simulink model "dyn_ESM_KF_SSM_VI_data"  (R2024b)
settings: Solver=ode1be  StartTime=0.0  StopTime=10  FixedStep=0.001  RelTol=1e-3
values from neighbouring files (symbols this model uses):
  A = [a11 a12; a21 a22]    [bicycleModelParam.m]
  B = [b1; b2]    [bicycleModelParam.m]
  H = [1 0;0 1]    [bicycleModelParam.m]
  Q = diag([0.2, 0.2, 0.01, 0.5, 0.3, 0.0001, 0.001, 0, 0.05])    [Copy_of_bicycleModelParam.m]    (also in bicycleModelParam.m = [0.8 0.2; 0.4 0.8])
  R = 0.001    [bicycleModelParam.m]
  v = 18/3.6    (= 5)    [bicycleModelParam.m]
libraries: simulink_extras x10
settings Model: Creator=fanny  LastModifiedBy=fanny
settings OptimizationCC: BlockReduction=off  DefaultParameterBehavior=Inlined  BufferReuse=off
settings DebuggingCC: AlgebraicLoopMsg=none

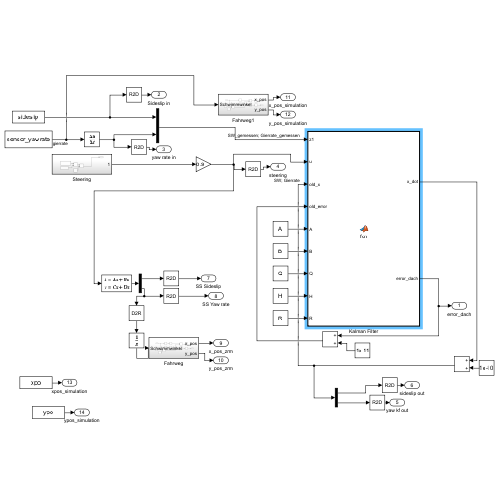
[thumbnail: Simulink's stored preview of the top-level diagram]
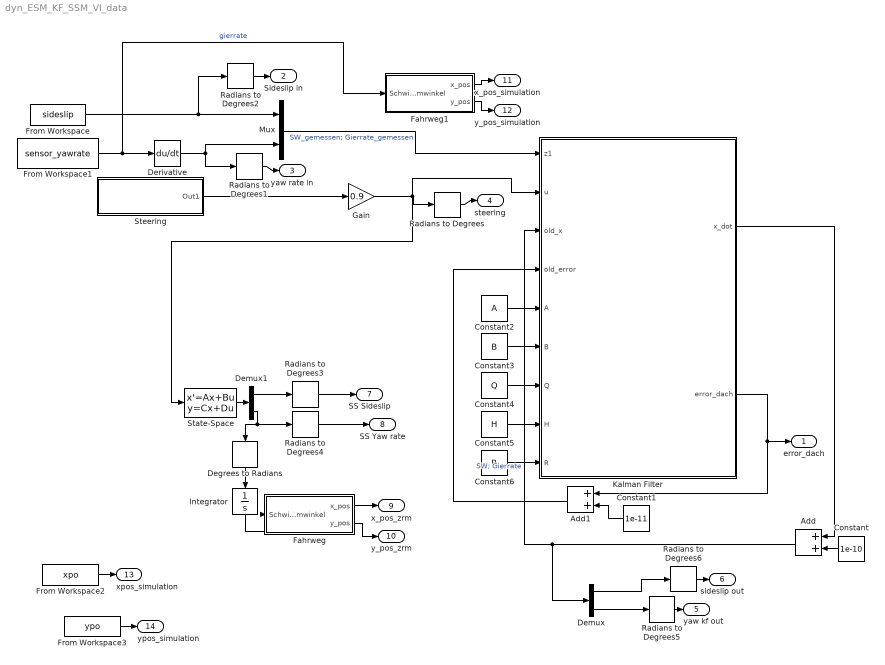
== system dyn_ESM_KF_SSM_VI_data ==
  Add : Sum
  Add1 : Sum
  Constant : Constant  Value=1e-10
  Constant1 : Constant  Value=1e-11
  Constant2 : Constant  Value=A
  Constant3 : Constant  Value=B
  Constant4 : Constant  Value=Q
  Constant5 : Constant  Value=H
  Constant6 : Constant  Value=R
  Degrees to Radians : simulink_extras/Transformations/Degrees to Radians
  Demux : Demux  Outputs=2
  Demux1 : Demux  Outputs=2
  Derivative : Derivative
  Fahrweg : Subsystem
  Fahrweg1 : Subsystem
  From Workspace : FromWorkspace  VariableName=sideslip
  From Workspace1 : FromWorkspace  VariableName=sensor_yawrate
  From Workspace2 : FromWorkspace  VariableName=xpo
  From Workspace3 : FromWorkspace  VariableName=ypo
  Gain : Gain  Gain=0.9
  Integrator : Integrator
  Kalman Filter : MATLAB Function  TreatAsAtomicUnit=on
  Mux : Mux  Inputs=2
  Radians to Degrees{,1..6} (7 alike) : simulink_extras/Transformations/Radians to Degrees
  State-Space : StateSpace  A=A  B=B  C=[1 0; 0 57]  D=[0; 0]  InitialCondition=0
  Steering : Subsystem
  error_dach : Outport
  Sideslip in : Outport  Port=2
  yaw rate in : Outport  Port=3
  steering : Outport  Port=4
  yaw kf out : Outport  Port=5
  sideslip out : Outport  Port=6
  SS Sideslip : Outport  Port=7
  SS Yaw rate : Outport  Port=8
  x_pos_zrm : Outport  Port=9
  y_pos_zrm : Outport  Port=10
  x_pos_simulation : Outport  Port=11
  y_pos_simulation : Outport  Port=12
  xpos_simulation : Outport  Port=13
  ypos_simulation : Outport  Port=14
  wires:
  Add1/1 -> Kalman Filter/4(old_error)
  Constant3/1 -> Kalman Filter/6(B)
  Mux/1 -> Kalman Filter/1(z1)  "SW_gemessen; Gierrate_gemessen"
  Constant/1 -> Add/2
  Kalman Filter/1(x_dot) -> Add/1
  Add/1 -> Kalman Filter/3(old_x), Demux/1  "SW; Gierrate"
  Constant2/1 -> Kalman Filter/5(A)
  Kalman Filter/2(error_dach) -> Add1/1, error_dach/1
  Constant1/1 -> Add1/2
  Constant4/1 -> Kalman Filter/7(Q)
  Constant5/1 -> Kalman Filter/8(H)
  Constant6/1 -> Kalman Filter/9(R)
  Demux/1 -> Radians to Degrees6/1
  Demux/2 -> Radians to Degrees5/1
  State-Space/1 -> Demux1/1
  Steering/1(Out1) -> Gain/1
  Radians to Degrees/1 -> steering/1
  From Workspace1/1 -> Fahrweg1/1(Schwimmwinkel), Derivative/1  "gierrate"
  Radians to Degrees1/1 -> yaw rate in/1
  Radians to Degrees2/1 -> Sideslip in/1
  Demux1/1 -> Radians to Degrees3/1
  Radians to Degrees6/1 -> sideslip out/1
  Radians to Degrees5/1 -> yaw kf out/1
  Derivative/1 -> Mux/2, Radians to Degrees1/1
  Fahrweg/2(y_pos) -> y_pos_zrm/1
  Fahrweg/1(x_pos) -> x_pos_zrm/1
  Fahrweg1/2(y_pos) -> y_pos_simulation/1
  Fahrweg1/1(x_pos) -> x_pos_simulation/1
  From Workspace/1 -> Radians to Degrees2/1, Mux/1
  From Workspace2/1 -> xpos_simulation/1
  From Workspace3/1 -> ypos_simulation/1
  Radians to Degrees3/1 -> SS Sideslip/1
  Radians to Degrees4/1 -> SS Yaw rate/1
  Integrator/1 -> Fahrweg/1(Schwimmwinkel)
  Demux1/2 -> Radians to Degrees4/1, Degrees to Radians/1
  Degrees to Radians/1 -> Integrator/1
  Gain/1 -> State-Space/1, Radians to Degrees/1, Kalman Filter/2(u)

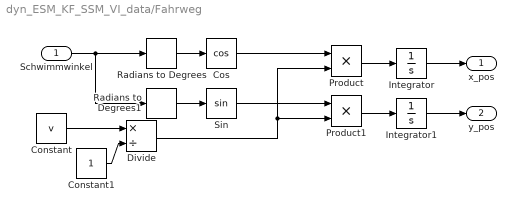
== system dyn_ESM_KF_SSM_VI_data/Fahrweg ==
  Schwimmwinkel : Inport
  Constant : Constant  Value=v
  Constant1 : Constant
  Cos : Trigonometry  Operator=cos
  Divide : Product  Inputs=*/
  Integrator : Integrator
  Integrator1 : Integrator
  Product : Product
  Product1 : Product
  Radians to Degrees : simulink_extras/Transformations/Radians to Degrees
  Radians to Degrees1 : simulink_extras/Transformations/Radians to Degrees
  Sin : Trigonometry
  x_pos : Outport
  y_pos : Outport  Port=2
  wires:
  Schwimmwinkel/1 -> Radians to Degrees1/1, Radians to Degrees/1
  Constant/1 -> Divide/1
  Cos/1 -> Product/1
  Product/1 -> Integrator/1
  Sin/1 -> Product1/1
  Product1/1 -> Integrator1/1
  Integrator/1 -> x_pos/1
  Integrator1/1 -> y_pos/1
  Divide/1 -> Product1/2, Product/2
  Constant1/1 -> Divide/2
  Radians to Degrees/1 -> Cos/1
  Radians to Degrees1/1 -> Sin/1

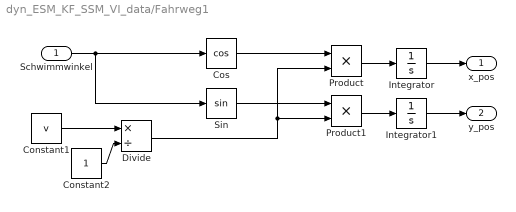
== system dyn_ESM_KF_SSM_VI_data/Fahrweg1 ==
  Schwimmwinkel : Inport
  Constant1 : Constant  Value=v
  Constant2 : Constant
  Cos : Trigonometry  Operator=cos
  Divide : Product  Inputs=*/
  Integrator : Integrator
  Integrator1 : Integrator
  Product : Product
  Product1 : Product
  Sin : Trigonometry
  x_pos : Outport
  y_pos : Outport  Port=2
  wires:
  Schwimmwinkel/1 -> Sin/1, Cos/1
  Cos/1 -> Product/1
  Product/1 -> Integrator/1
  Sin/1 -> Product1/1
  Product1/1 -> Integrator1/1
  Integrator/1 -> x_pos/1
  Integrator1/1 -> y_pos/1
  Divide/1 -> Product1/2, Product/2
  Constant2/1 -> Divide/2
  Constant1/1 -> Divide/1

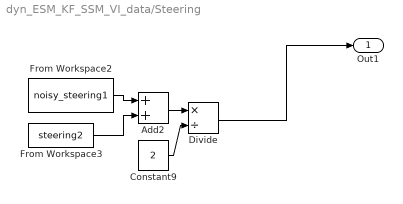
== system dyn_ESM_KF_SSM_VI_data/Steering ==
  Add2 : Sum
  Constant9 : Constant  Value=2
  Divide : Product  Inputs=*/
  From Workspace2 : FromWorkspace  VariableName=noisy_steering1
  From Workspace3 : FromWorkspace  VariableName=steering2
  Out1 : Outport
  wires:
  From Workspace3/1 -> Add2/2
  Constant9/1 -> Divide/2
  Divide/1 -> Out1/1
  From Workspace2/1 -> Add2/1
  Add2/1 -> Divide/1

== matlab function dyn_ESM_KF_SSM_VI_data/Kalman Filter ==
  data: z1 input; u input; x_dot output; old_x input; old_error input; error_dach output; A input; B input; Q input; H input; R input
function [x_dot, error_dach] = fcn(z1, u, old_x, old_error, A, B, Q, H, R)
% z1    : simulierte Sensordaten [beta, phi_punkt]
% u     : Lenkwinkel (rad)
% old_x : Vorheriger geschätzter Zustand
% oldErr: Vorherige Fehlerkovarianzmatrix
% A     : Zustandsübergangsmatrix 


% Vorhersageschritt 
x_pred = A * old_x + B * u; 
P_pred = A * old_error * A' + Q;   % Vorhergesagte Fehlerkovarianz
% Kalman-Gain Berechnung (Kalman Gain calculation)

up = P_pred * H';         
dwn = H * P_pred * H' + R;  
K_gain = up / dwn;

x_est = x_pred + K_gain * (z1 - H * x_pred);
P_est = (H - K_gain * H) * P_pred;      % Aktualisierte Fehlerkovarianz

x_dot = x_est(:,1);% x_est(2,1);  % Matrix 2x1 
error_dach = P_est;
